simulink model "pso_lqr_test"  (R2022b)
settings: Solver=VariableStepAuto  StartTime=0.0  StopTime=10.0  RelTol=1e-3
settings Model: Creator=bu  LastModifiedBy=bu

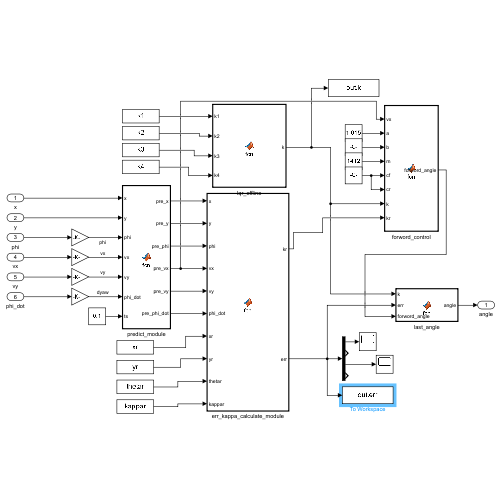
[thumbnail: Simulink's stored preview of the top-level diagram]
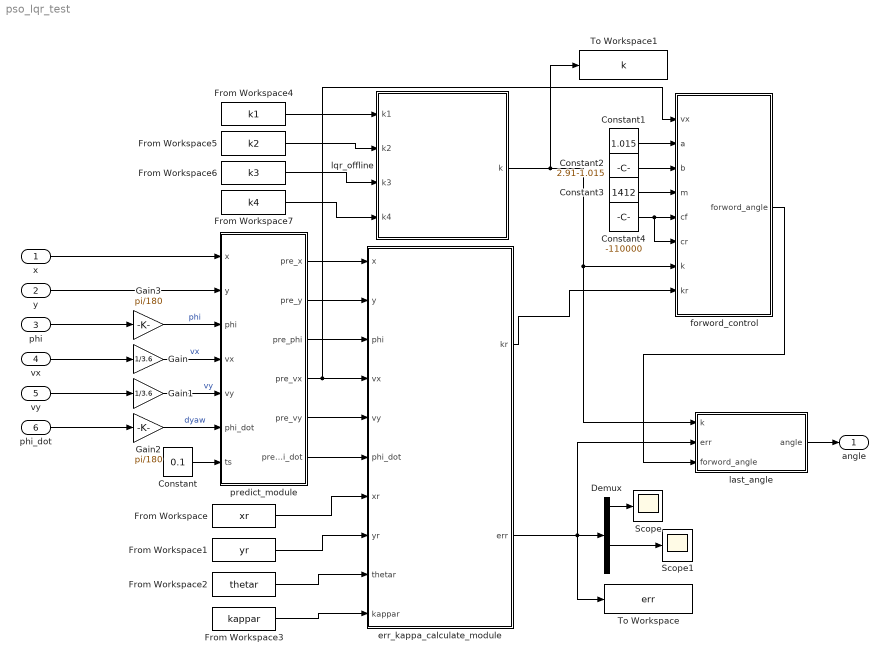
== system pso_lqr_test ==
  x : Inport
  y : Inport  Port=2
  phi : Inport  Port=3
  vx : Inport  Port=4
  vy : Inport  Port=5
  phi_dot : Inport  Port=6
  Constant : Constant  Value=0.1
  Constant1 : Constant  Value=1.015
  Constant2 : Constant  Value=2.91-1.015
  Constant3 : Constant  Value=1412
  Constant4 : Constant  Value=-110000
  Demux : Demux
  From Workspace : FromWorkspace  VariableName=xr  SampleTime=0.1
  From Workspace1 : FromWorkspace  VariableName=yr  SampleTime=0.1
  From Workspace2 : FromWorkspace  VariableName=thetar  SampleTime=0.1
  From Workspace3 : FromWorkspace  VariableName=kappar  SampleTime=0.1
  From Workspace4 : FromWorkspace  VariableName=k1
  From Workspace5 : FromWorkspace  VariableName=k2
  From Workspace6 : FromWorkspace  VariableName=k3
  From Workspace7 : FromWorkspace  VariableName=k4
  Gain : Gain  Gain=1/3.6
  Gain1 : Gain  Gain=1/3.6
  Gain2 : Gain  Gain=pi/180
  Gain3 : Gain  Gain=pi/180
  Scope : Scope
  Scope1 : Scope
  To Workspace : ToWorkspace  VariableName=err  SaveFormat=Timeseries  SampleTime=-1
  To Workspace1 : ToWorkspace  VariableName=k  SaveFormat=Timeseries  SampleTime=-1
  err_kappa_calculate_module : MATLAB Function  TreatAsAtomicUnit=on
  forword_control : MATLAB Function  TreatAsAtomicUnit=on
  last_angle : MATLAB Function  TreatAsAtomicUnit=on
  lqr_offline : MATLAB Function  TreatAsAtomicUnit=on
  predict_module : MATLAB Function  TreatAsAtomicUnit=on
  angle : Outport  VectorParamsAs1DForOutWhenUnconnected=off
  wires:
  Constant/1 -> predict_module/7(ts)
  phi/1 -> Gain3/1
  Constant4/1 -> forword_control/6(cr), forword_control/5(cf)
  From Workspace4/1 -> lqr_offline/1(k1)
  phi_dot/1 -> Gain2/1
  predict_module/5(pre_vy) -> err_kappa_calculate_module/5(vy)
  last_angle/1(angle) -> angle/1
  Gain2/1 -> predict_module/6(phi_dot)  "dyaw"
  vy/1 -> Gain1/1
  predict_module/6(pre_phi_dot) -> err_kappa_calculate_module/6(phi_dot)
  Gain3/1 -> predict_module/3(phi)  "phi"
  forword_control/1(forword_angle) -> last_angle/3(forword_angle)
  predict_module/1(pre_x) -> err_kappa_calculate_module/1(x)
  err_kappa_calculate_module/1(kr) -> forword_control/8(kr)
  Constant2/1 -> forword_control/3(b)
  Gain/1 -> predict_module/4(vx)  "vx"
  predict_module/2(pre_y) -> err_kappa_calculate_module/2(y)
  y/1 -> predict_module/2(y)
  From Workspace6/1 -> lqr_offline/3(k3)
  Constant3/1 -> forword_control/4(m)
  vx/1 -> Gain/1
  err_kappa_calculate_module/2(err) -> Demux/1, To Workspace/1, last_angle/2(err)
  From Workspace7/1 -> lqr_offline/4(k4)
  Gain1/1 -> predict_module/5(vy)  "vy"
  predict_module/3(pre_phi) -> err_kappa_calculate_module/3(phi)
  From Workspace5/1 -> lqr_offline/2(k2)
  predict_module/4(pre_vx) -> forword_control/1(vx), err_kappa_calculate_module/4(vx)
  lqr_offline/1(k) -> To Workspace1/1, last_angle/1(k), forword_control/7(k)
  Constant1/1 -> forword_control/2(a)
  x/1 -> predict_module/1(x)
  From Workspace3/1 -> err_kappa_calculate_module/10(kappar)
  From Workspace2/1 -> err_kappa_calculate_module/9(thetar)
  From Workspace1/1 -> err_kappa_calculate_module/8(yr)
  From Workspace/1 -> err_kappa_calculate_module/7(xr)
  Demux/1 -> Scope/1
  Demux/3 -> Scope1/1

== matlab function pso_lqr_test/err_kappa_calculate_module ==
  data: x input; kr output; y input; phi input; vx input; vy input; phi_dot input; xr input; yr input; thetar input; kappar input; err output
function [kr,err] = fcn(x,y,phi,vx,vy,phi_dot,xr,yr,thetar,kappar)
    n=length(xr);
    d_min=(x-xr(1))^2+(y-yr(1))^2;
    min=1;
    for i=1:n
        d=(x-xr(i))^2+(y-yr(i))^2;
        if d<d_min
            d_min=d;
            min=i;
        end
    end
    dmin=min;
    tor=[cos(thetar(dmin));sin(thetar(dmin))];
    nor=[-sin(thetar(dmin));cos(thetar(dmin))];
    d_err=[x-xr(dmin);y-yr(dmin)];
    ed=nor'*d_err;
    es=tor'*d_err;
    %projection_point_thetar=thetar(dmin);%apollo
    projection_point_thetar=thetar(dmin)+kappar(dmin)*es;
    ed_dot=vy*cos(phi-projection_point_thetar)+vx*sin(phi-projection_point_thetar);
    %%%%%%%%%
    ephi=sin(phi-projection_point_thetar);
    %因为在推导假设了ephi是小角度（锐角），且角度具有多值性，用sin来解决
    %%%%%%%%%
    s_dot=vx*cos(phi-projection_point_thetar)-vy*sin(phi-projection_point_thetar);
    s_dot=s_dot/(1-kappar(dmin)*ed);
    ephi_dot=phi_dot-kappar(dmin)*s_dot;
    kr=kappar(dmin);
    err=[ed;ed_dot;ephi;ephi_dot];
    
  

end

== matlab function pso_lqr_test/predict_module ==
  data: x input; pre_x output; y input; phi input; vx input; vy input; phi_dot input; pre_y output; pre_phi output; pre_vx output; pre_vy output; pre_phi_dot output; ts input
function [pre_x,pre_y,pre_phi,pre_vx,pre_vy,pre_phi_dot] = fcn(x,y,phi,vx,vy,phi_dot,ts)
    pre_x=x+vx*ts*cos(phi)-vy*ts*sin(phi);
    pre_y=y+vy*ts*cos(phi)+vx*ts*sin(phi);
    pre_phi=phi+phi_dot*ts;
    pre_vx=vx;
    pre_vy=vy;
    pre_phi_dot=phi_dot;
end

== matlab function pso_lqr_test/lqr_offline ==
  data: k1 input; k output; k2 input; k3 input; k4 input
function k  = fcn(k1,k2,k3,k4)
    k1 = [k1,k2,k3,k4];
    k = [;k1];
end

== matlab function pso_lqr_test/forword_control ==
  data: vx input; a input; forword_angle output; b input; m input; cf input; cr input; k input; kr input
function forword_angle = fcn(vx,a,b,m,cf,cr,k,kr)
    forword_angle=kr*(a+b-b*k(3)-(m*vx*vx/(a+b))*((b/cf)+(a/cr)*k(3)-(a/cr)));
end

== matlab function pso_lqr_test/last_angle ==
  data: k input; angle output; err input; forword_angle input
function angle = fcn(k,err,forword_angle)

    angle=-k*err+forword_angle;
end
